simulink model "Project2_Trial2"  (R2023b)
settings: Solver=VariableStepAuto  StartTime=0.0  StopTime=10.0  RelTol=1e-3
values from neighbouring files (symbols this model uses):
  A = 3    [Project2_Trial2.m]
  F = 2    [Project2_Trial2.m]
  Ti = 0.5    [Project2_Trial2.m]
settings Model: Creator=mfb36  LastModifiedBy=mfb36

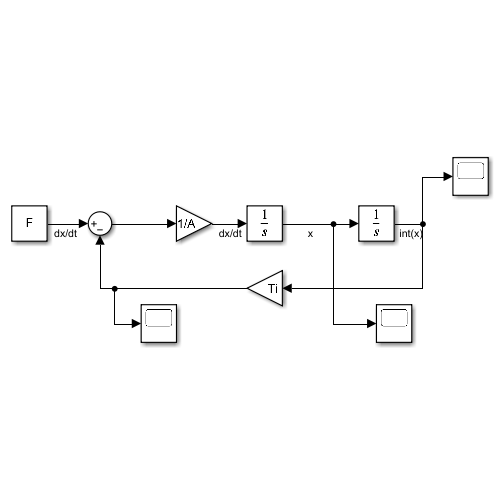
[thumbnail: Simulink's stored preview of the top-level diagram]
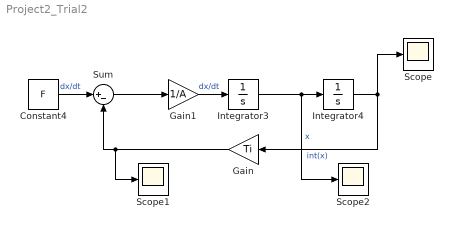
== system Project2_Trial2 ==
  Constant4 : Constant  Value=F
  Gain : Gain  Gain=Ti
  Gain1 : Gain  Gain=1/A
  Integrator3 : Integrator
  Integrator4 : Integrator
  Scope : Scope
  Scope1 : Scope
  Scope2 : Scope
  Sum : Sum  Inputs=|+-
  wires:
  Gain/1 -> Scope1/1, Sum/2
  Sum/1 -> Gain1/1
  Integrator3/1 -> Scope2/1, Integrator4/1  "x"
  Constant4/1 -> Sum/1  "dx/dt"
  Gain1/1 -> Integrator3/1  "dx/dt"
  Integrator4/1 -> Gain/1, Scope/1  "int(x)"
